simulink model "rocketSim"  (R2019a)
settings: Solver=ode3  StartTime=0.0  StopTime=t2  FixedStep=simPrm.h  MaxStep=simPrm.h  RelTol=1e-3
undefined symbols (not defined in the file or in its folder): thr
libraries: sm_lib x6, nesl_utility x6, simulink_extras x2
settings Model: Creator=vmali  LastModifiedBy=vmali
settings DebuggingCC: BusObjectLabelMismatch=none
settings SimscapeCC: SimscapeNormalizeSystem=off  SimscapeLogType=all
settings ExplorerConfigSet: InternalSimMechanicsExplorerSettings="<ExplorerConfiguration><canonicalview>default</canonicalview><AnimationSetting><BasePlaybackSpeed>1.0</BasePlaybackSpeed><PlaybackSpeedFactor>1.0</PlaybackSpeedFactor></AnimationSetting><TilePanel><TileInfo><Tiles Columns=\"1\" Count=\"1\" Rows=\"1\"><Column Weight=\"1\"/><Row Weight=\"1\"/><Tile Height=\"1\" Width=\"1\" X=\"0\" Y=\"0\"/></Tiles></TileInfo><SceneInfo><SceneViewer><BGColor><R>0.60000002384185791</R><G>0.60000002384185791</G><B>0.60000002384185791</B></BGColor><Camera><DoPerspective>off</DoPerspective><Position><X>172.69681181507903</X><Y>-34.9970129098614251</Y><Z>180.545841253777326</Z></Position><Center><X>172.518361402320892</X><Y>-34.4223760725900263</Y><Z>0.262351084401639012</Z></Center><Up><X>-0.00981184985509124183</X><Y>0.999946752141307016</Y><Z>0.00319694924480169555</Z></Up><ViewLimDist>1</ViewLimDist><YLim>132.755471146486911</YLim><XLim>205.915521409793769</XLim></Camera></SceneViewer></SceneInfo></TilePanel><MechEditorPanel><Cameras/><GfxPanelCameraMap/><VideoCreator><PlaybackSpeedRatio>1.0</PlaybackSpeedRatio><FrameRate>30</FrameRate><VideoFormat>Motion JPEG AVI</VideoFormat><FrameSize>auto</FrameSize></VideoCreator></MechEditorPanel></ExplorerConfiguration>"

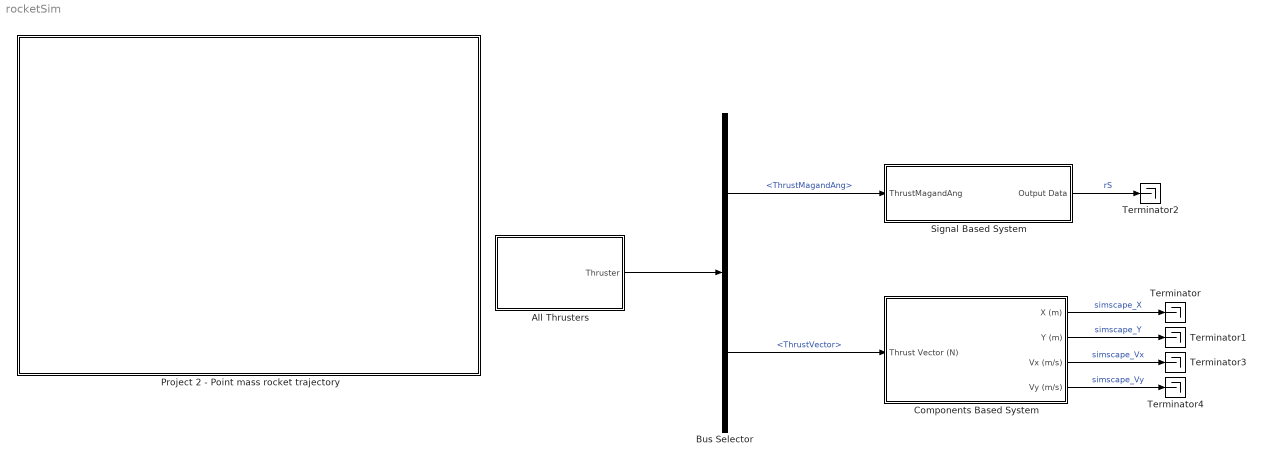
== system rocketSim ==
  All Thrusters : Subsystem
  Bus Selector : BusSelector  OutputSignals=ThrustMagandAng,ThrustVector
  Components Based System : Subsystem
  Project 2 - Point mass rocket trajectory : Subsystem
      mask Display:
      | % Use specified image as mask icon
      | image('Project2.jpg')
  Signal Based System : Subsystem
  Terminator{,1..4} (5 alike) : Terminator
  wires:
  All Thrusters/1(Thruster) -> Bus Selector/1
  Bus Selector/2 -> Components Based System/1(Thrust Vector (N))  "<ThrustVector>"
  Components Based System/1(X (m)) -> Terminator/1  "simscape_X"
  Components Based System/2(Y (m)) -> Terminator1/1  "simscape_Y"
  Bus Selector/1 -> Signal Based System/1(ThrustMagandAng)  "<ThrustMagandAng>"
  Signal Based System/1(Output Data) -> Terminator2/1  "rS"
  Components Based System/3(Vx (m/s)) -> Terminator3/1  "simscape_Vx"
  Components Based System/4(Vy (m/s)) -> Terminator4/1  "simscape_Vy"

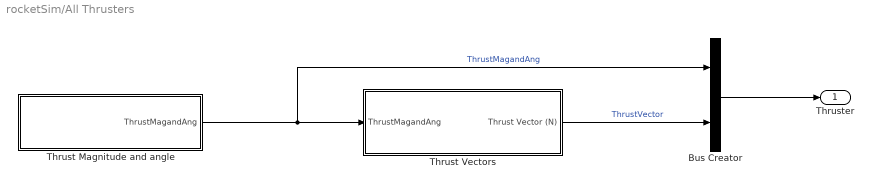
== system rocketSim/All Thrusters ==
  Bus Creator : BusCreator  Inputs=2
  Thrust Magnitude and angle : Subsystem  Variant=on
  Thrust Vectors : Subsystem
  Thruster : Outport
  wires:
  Bus Creator/1 -> Thruster/1
  Thrust Vectors/1(Thrust Vector (N)) -> Bus Creator/2  "ThrustVector"
  Thrust Magnitude and angle/1(ThrustMagandAng) -> Thrust Vectors/1(ThrustMagandAng), Bus Creator/1  "ThrustMagandAng"

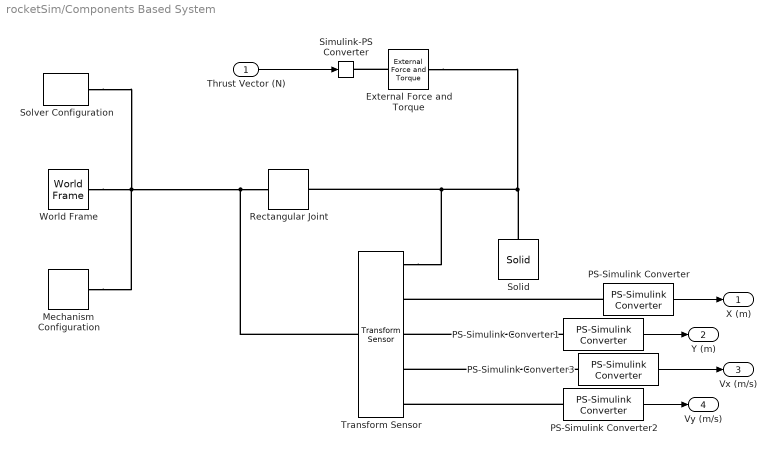
== system rocketSim/Components Based System ==
  Thrust Vector (N) : Inport
  External Force and Torque : sm_lib/Forces and Torques/External Force and Torque  ForceResolutionFrame=AttachedFrame  EnableForceX=off  EnableForceY=off  EnableForceZ=off  EnableForce=on  TorqueResolutionFrame=AttachedFrame  EnableTorqueX=off  EnableTorqueY=off  EnableTorqueZ=off  EnableTorque=off
  Mechanism Configuration : sm_lib/Utilities/Mechanism Configuration  UniformGravity=Constant  GravityVector=[0 -10.0 0]  GravityUnits=m/s^2  LinearizationDelta=0.001
  PS-Simulink Converter{,1..3} (4 alike) : nesl_utility/PS-Simulink Converter  PhysicalDomain=network_engine_domain  SubClassName=ps_output  LeftPortType=input  RightPortType=output  PseudoPeriodic=off  Frequencies=[]  Unit=1  AffineConversion=off
  Rectangular Joint : sm_lib/Joints/Rectangular Joint  SenseConstraintForce=off  SenseConstraintForceX=off  SenseConstraintForceY=off  SenseConstraintForceZ=off  SenseConstraintTorque=off  SenseConstraintTorqueX=off  SenseConstraintTorqueY=off  SenseConstraintTorqueZ=off  SenseTotalForce=off  SenseTotalForceX=off  SenseTotalForceY=off  SenseTotalForceZ=off  SenseTotalTorque=off  SenseTotalTorqueX=off  SenseTotalTorqueY=off  SenseTotalTorqueZ=off  CompositeWrenchDir=FollowerOnBase  CompositeWrenchFrame=BaseFrame  PxEquilibriumPosition=0  PxEquilibriumPositionUnits=m  PxSpringStiffness=0  PxSpringStiffnessUnits=N/m  PxDampingCoefficient=0  PxDampingCoefficientUnits=N/(m/s)  PxTorqueActuationMode=NoTorque  PxMotionActuationMode=ComputedMotion  PxSensePosition=off  PxSenseVelocity=off  PxSenseAcceleration=off  PxSenseTorqueForce=off  PxSenseLowerLimitTorqueForce=off  PxSenseUpperLimitTorqueForce=off  PxLowerLimitSpecify=off  PxLowerLimitBound=-1  PxLowerLimitBoundUnits=m  PxLowerLimitStiffness=1e6  PxLowerLimitStiffnessUnits=N/m  PxLowerLimitDamping=1e3  PxLowerLimitDampingUnits=N/(m/s)  PxLowerLimitTransitionRegionWidth=1e-4  PxLowerLimitTransitionRegionWidthUnits=m  PxUpperLimitSpecify=off  PxUpperLimitBound=1  PxUpperLimitBoundUnits=m  PxUpperLimitStiffness=1e6  PxUpperLimitStiffnessUnits=N/m  PxUpperLimitDamping=1e3  PxUpperLimitDampingUnits=N/(m/s)  PxUpperLimitTransitionRegionWidth=1e-4  PxUpperLimitTransitionRegionWidthUnits=m  PxPositionTargetSpecify=off  PxPositionTargetPriority=High  PxPositionTargetValue=0  PxPositionTargetValueUnits=m  PxVelocityTargetSpecify=off  PxVelocityTargetPriority=High  PxVelocityTargetValue=0  PxVelocityTargetValueUnits=m/s  PyEquilibriumPosition=0  PyEquilibriumPositionUnits=m  PySpringStiffness=0  PySpringStiffnessUnits=N/m  PyDampingCoefficient=0  PyDampingCoefficientUnits=N/(m/s)  PyTorqueActuationMode=NoTorque  PyMotionActuationMode=ComputedMotion  PySensePosition=off  PySenseVelocity=off  PySenseAcceleration=off  PySenseTorqueForce=off  PySenseLowerLimitTorqueForce=off  PySenseUpperLimitTorqueForce=off  PyLowerLimitSpecify=off  PyLowerLimitBound=-1  PyLowerLimitBoundUnits=m  PyLowerLimitStiffness=1e6  PyLowerLimitStiffnessUnits=N/m  PyLowerLimitDamping=1e3  PyLowerLimitDampingUnits=N/(m/s)  PyLowerLimitTransitionRegionWidth=1e-4  PyLowerLimitTransitionRegionWidthUnits=m  PyUpperLimitSpecify=off  PyUpperLimitBound=1  PyUpperLimitBoundUnits=m  PyUpperLimitStiffness=1e6  PyUpperLimitStiffnessUnits=N/m  PyUpperLimitDamping=1e3  PyUpperLimitDampingUnits=N/(m/s)  PyUpperLimitTransitionRegionWidth=1e-4  PyUpperLimitTransitionRegionWidthUnits=m  PyPositionTargetSpecify=off  PyPositionTargetPriority=High  PyPositionTargetValue=0  PyPositionTargetValueUnits=m  PyVelocityTargetSpecify=off  PyVelocityTargetPriority=High  PyVelocityTargetValue=0  PyVelocityTargetValueUnits=m/s
      settings: SourceProductName=Simscape Multibody
  Simulink-PS Converter : nesl_utility/Simulink-PS Converter  PhysicalDomain=network_engine_domain  SubClassName=ps_input  LeftPortType=input  RightPortType=output  PseudoPeriodic=off  Frequencies=[]  NoiseDistribution=none  NoiseParameters=[]  Unit=1  AffineConversion=off  FilteringAndDerivatives=provide  SimscapeFilterOrder=1  InputFilterTimeConstant=0.001  UdotUserProvided=0
  Solid : sm_lib/Body Elements/Solid  InertiaType=PointMass  Mass=1000  MassUnits=kg  CenterOfMass=[0 0 0]  CenterOfMassUnits=m  MomentsOfInertia=[1 1 1]  MomentsOfInertiaUnits=kg*m^2  ProductsOfInertia=[0 0 0]  ProductsOfInertiaUnits=kg*m^2  BasedOnType=Density  Density=1000  DensityUnits=kg/m^3  DoExposeReferenceFrame=on  SerializedFrames=<Frames/>  GraphicType=FromGeometry  MarkerShape=Sphere  MarkerSize=10  GraphicVisPropType=SimpleVisualProperties  GraphicDiffuseColor=[1.0 0.2 0.2]  GraphicSpecularColor=[0.5 0.5 0.5 1.0]  GraphicAmbientColor=[0.15 0.15 0.15 1.0]  GraphicEmissiveColor=[0.0 0.0 0.0 1.0]  GraphicShininess=75  GraphicOpacity=1.0  GeometryShape=Sphere  RectangleSize=[1 1]  RectangleSizeUnits=m  BrickDimensions=[1 1 1]  BrickDimensionUnits=m  CylinderRadius=1  CylinderRadiusUnits=m  CylinderLength=1  CylinderLengthUnits=m  SphereRadius=1  SphereRadiusUnits=m  EllipsoidRadii=[1 1 1]  EllipsoidRadiiUnits=m  ExtrusionCrossSection=[1 1; -1 1; -1 -1; 1 -1]  ExtrusionCrossSectionUnits=m  ExtrusionLength=1  ExtrusionLengthUnits=m  PolygonNumSides=3  PolygonOuterRadius=1  PolygonOuterRadiusUnits=m  ExtGeomFileType=STEP  ExtGeomFileUnits=m  RevolutionCrossSection=[1 1; 1 -1; 2 -1; 2 1]  RevolutionCrossSectionUnits=m  RevolutionExtent=Full  RevolutionAngle=180  RevolutionAngleUnits=deg
  Solver Configuration : nesl_utility/Solver Configuration  PhysicalDomain=network_engine_domain  SubClassName=solver  LeftPortType=input  RightPortType=generic  Tones=[]  Harmonics=[]  SimulateNoise=off  Profile=off  UseLocalSampling=off  EnableSwitchedLinearOptims=on  FrequencyDomain=off  UseCCode=off  RelTol=0.001  AbsTol=1e-06  MinStep=1e-09  ToWorkspace=off  RevertToSquareIcSolve=off  NumHomotopyIterations=100  PhasorMode=off  PhasorModeNumHarmonics=1  DoDC=off  ResidualTolerance=1e-09  UseLocalSolver=off  LocalSolverChoice=NE_BACKWARD_EULER_ADVANCER  LocalSolverSampleTime=0.001  DoFixedCost=off  MaxNonlinIter=3  MaxModeIter=2  LinearAlgebra=auto  EquationFormulation=NE_TIME_EF  DelaysMemoryBudget=1024  AutomaticFiltering=on  FilteringTimeConstant=0.001  PartitionStorageMethod=AS_NEEDED  PartitionMemoryBudget=1024  PartitionMethod=ROBUST
  Transform Sensor : sm_lib/Frames and Transforms/Transform Sensor  MeasurementFrame=World  SenseAngle=off  SenseAxis=off  SenseAngle1=off  SenseAngle2=off  SenseAngle3=off  SenseQ=off  SenseR=off  SenseOmegaX=off  SenseOmegaY=off  SenseOmegaZ=off  SenseOmega1=off  SenseOmega2=off  SenseOmega3=off  SenseQDot=off  SenseRDot=off  SenseAlphaX=off  SenseAlphaY=off  SenseAlphaZ=off  SenseAlpha1=off  SenseAlpha2=off  SenseAlpha3=off  SenseQDDot=off  SenseRDDot=off  SenseX=on  SenseY=on  SenseZ=off  SenseRad=off  SenseAzim=off  SenseDist=off  SenseInc=off  SenseXDot=on  SenseYDot=on  SenseZDot=off  SenseRadDot=off  SenseAzimDot=off  SenseDistDot=off  SenseIncDot=off  SenseXDDot=off  SenseYDDot=off  SenseZDDot=off  SenseRadDDot=off  SenseAzimDDot=off  SenseDistDDot=off  SenseIncDDot=off
  World Frame : sm_lib/Frames and Transforms/World Frame
  X (m) : Outport
  Y (m) : Outport  Port=2
  Vx (m/s) : Outport  Port=3
  Vy (m/s) : Outport  Port=4
  wires:
  Thrust Vector (N)/1 -> Simulink-PS Converter/1
  PS-Simulink Converter/1 -> X (m)/1
  PS-Simulink Converter1/1 -> Y (m)/1
  PS-Simulink Converter2/1 -> Vy (m/s)/1
  PS-Simulink Converter3/1 -> Vx (m/s)/1
  connections:
  World Frame/RConn1 -- Mechanism Configuration/RConn1 -- Solver Configuration/RConn1 -- Transform Sensor/LConn1 -- Rectangular Joint/LConn1
  Solid/RConn1 -- External Force and Torque/RConn1 -- Transform Sensor/RConn1 -- Rectangular Joint/RConn1
  External Force and Torque/LConn1 -- Simulink-PS Converter/RConn1
  PS-Simulink Converter/LConn1 -- Transform Sensor/RConn2
  PS-Simulink Converter1/LConn1 -- Transform Sensor/RConn3
  PS-Simulink Converter2/LConn1 -- Transform Sensor/RConn5
  PS-Simulink Converter3/LConn1 -- Transform Sensor/RConn4

== system rocketSim/Project 2 - Point mass rocket trajectory ==

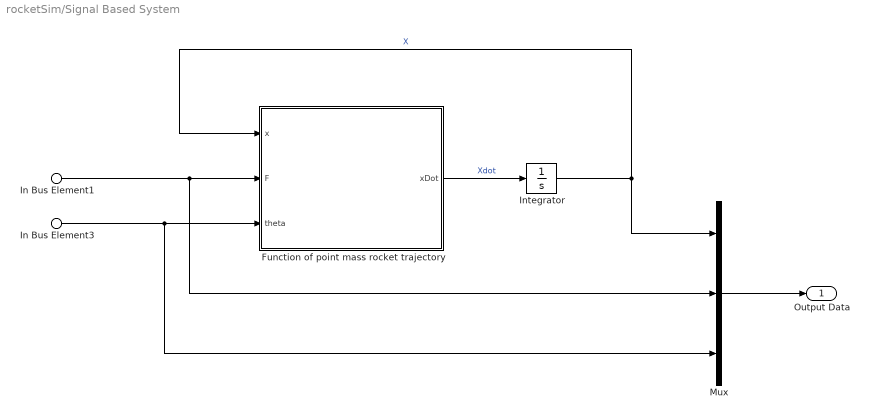
== system rocketSim/Signal Based System ==
  In Bus Element1 : Inport  PortName=ThrustMagandAng  Element=Magnitude
  In Bus Element3 : Inport  PortName=ThrustMagandAng  Element=Angle
  Function of point mass rocket trajectory : MATLAB Function  TreatAsAtomicUnit=on
  Integrator : Integrator
  Mux : Mux  Inputs=3
  Output Data : Outport
  wires:
  Function of point mass rocket trajectory/1(xDot) -> Integrator/1  "Xdot"
  Integrator/1 -> Mux/1, Function of point mass rocket trajectory/1(x)  "X"
  In Bus Element1/1 -> Mux/2, Function of point mass rocket trajectory/2(F)
  In Bus Element3/1 -> Mux/3, Function of point mass rocket trajectory/3(theta)
  Mux/1 -> Output Data/1

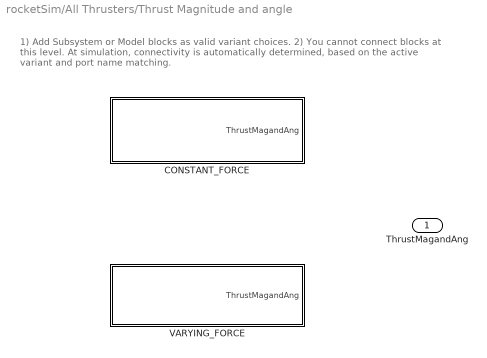
== system rocketSim/All Thrusters/Thrust Magnitude and angle ==
  note: 1) Add Subsystem or Model blocks as valid variant choices.
      | 2) You cannot connect blocks at this level. At simulation, connectivity is automatically
      | determined, based on the active variant and port name matching.
  CONSTANT_FORCE : Subsystem  Description=This is the block containing the constant thrust value.  VariantControl=CONSTANT_F_VSS
  VARYING_FORCE : Subsystem  Description=This is the block containing the constant thrust value.  VariantControl=VARYING_F_VSS
  ThrustMagandAng : Outport

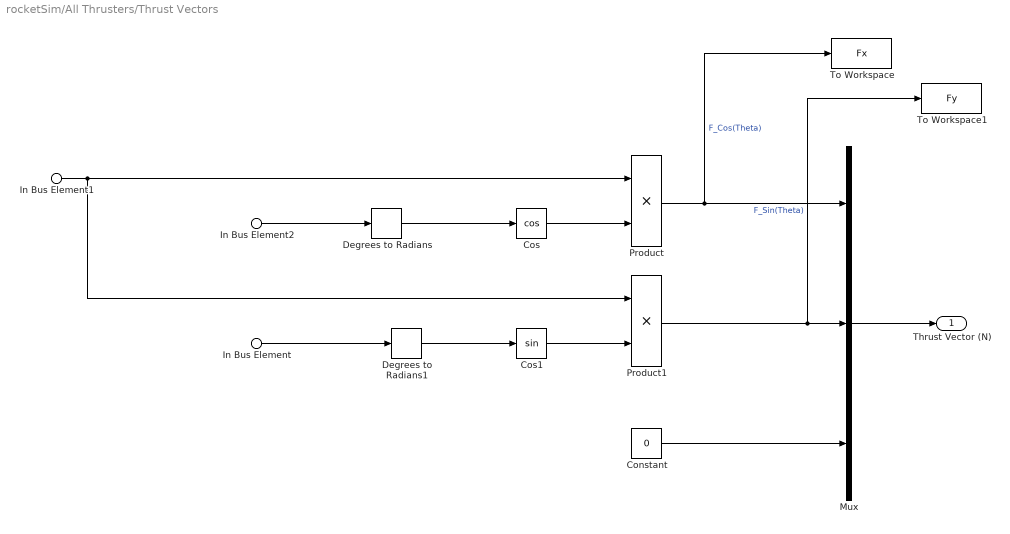
== system rocketSim/All Thrusters/Thrust Vectors ==
  In Bus Element1 : Inport  PortName=ThrustMagandAng  Element=Magnitude
  In Bus Element2 : Inport  PortName=ThrustMagandAng  Element=Angle
  In Bus Element : Inport  PortName=ThrustMagandAng  Element=Angle
  Constant : Constant  Value=0
  Cos : Trigonometry  Operator=cos
  Cos1 : Trigonometry
  Degrees to Radians : simulink_extras/Transformations/Degrees to Radians
  Degrees to Radians1 : simulink_extras/Transformations/Degrees to Radians
  Mux : Mux  Inputs=3
  Product : Product
  Product1 : Product
  To Workspace : ToWorkspace  VariableName=Fx  SaveFormat=Timeseries  SampleTime=-1
  To Workspace1 : ToWorkspace  VariableName=Fy  SaveFormat=Timeseries  SampleTime=-1
  Thrust Vector (N) : Outport
  wires:
  In Bus Element2/1 -> Degrees to Radians/1
  Cos/1 -> Product/2
  In Bus Element/1 -> Degrees to Radians1/1
  In Bus Element1/1 -> Product1/1, Product/1
  Cos1/1 -> Product1/2
  Product/1 -> To Workspace/1, Mux/1  "F_Cos(Theta)"
  Product1/1 -> To Workspace1/1, Mux/2  "F_Sin(Theta)"
  Constant/1 -> Mux/3
  Mux/1 -> Thrust Vector (N)/1
  Degrees to Radians/1 -> Cos/1
  Degrees to Radians1/1 -> Cos1/1

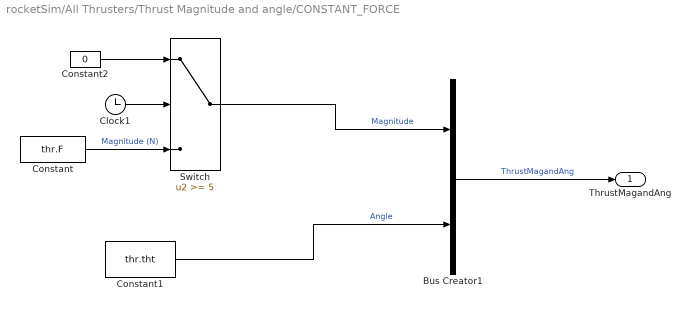
== system rocketSim/All Thrusters/Thrust Magnitude and angle/CONSTANT_FORCE ==
  Bus Creator1 : BusCreator  Inputs=2
  Clock1 : Clock
  Constant : Constant  Value=thr.F
  Constant1 : Constant  Value=thr.tht
  Constant2 : Constant  Value=0
  Switch : Switch  Threshold=5
  ThrustMagandAng : Outport  OutDataTypeStr=Bus: Scenario_1
  wires:
  Constant1/1 -> Bus Creator1/2  "Angle"
  Clock1/1 -> Switch/2
  Constant2/1 -> Switch/1
  Constant/1 -> Switch/3  "Magnitude (N)"
  Switch/1 -> Bus Creator1/1  "Magnitude"
  Bus Creator1/1 -> ThrustMagandAng/1  "ThrustMagandAng"

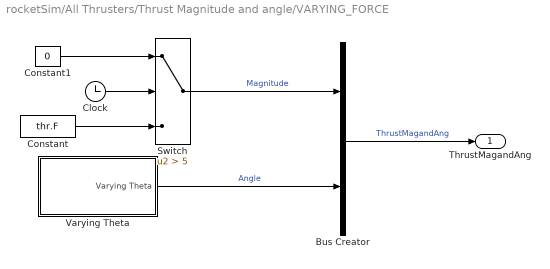
== system rocketSim/All Thrusters/Thrust Magnitude and angle/VARYING_FORCE ==
  Bus Creator : BusCreator  Inputs=2
  Clock : Clock
  Constant : Constant  Value=thr.F
  Constant1 : Constant  Value=0
  Switch : Switch  Criteria=u2 > Threshold  Threshold=5
  Varying Theta : Subsystem
  ThrustMagandAng : Outport  OutDataTypeStr=Bus: Scenario_2
  wires:
  Varying Theta/1(Varying Theta) -> Bus Creator/2  "Angle"
  Bus Creator/1 -> ThrustMagandAng/1  "ThrustMagandAng"
  Constant1/1 -> Switch/1
  Constant/1 -> Switch/3
  Switch/1 -> Bus Creator/1  "Magnitude"
  Clock/1 -> Switch/2

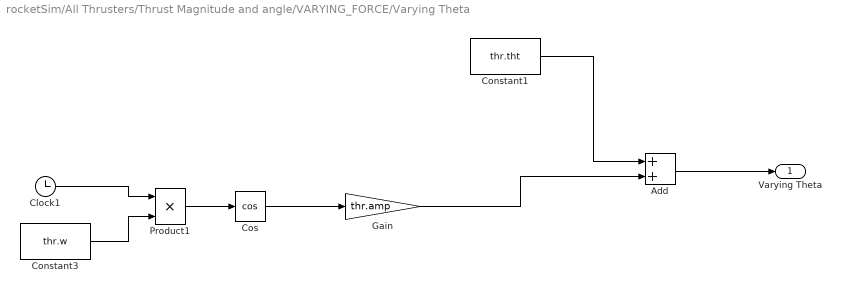
== system rocketSim/All Thrusters/Thrust Magnitude and angle/VARYING_FORCE/Varying Theta ==
  Add : Sum
  Clock1 : Clock
  Constant1 : Constant  Value=thr.tht
  Constant3 : Constant  Value=thr.w
  Cos : Trigonometry  Operator=cos
  Gain : Gain  Gain=thr.amp
  Product1 : Product
  Varying Theta : Outport
  wires:
  Gain/1 -> Add/2
  Constant1/1 -> Add/1
  Add/1 -> Varying Theta/1
  Product1/1 -> Cos/1
  Constant3/1 -> Product1/2
  Clock1/1 -> Product1/1
  Cos/1 -> Gain/1

== matlab function rocketSim/Signal Based System/Function of point mass rocket trajectory ==
  data: x input; xDot output; F input; theta input
function xDot = f(x,F, theta)
% Function f of x' = f(x)
% x == states

%Give the input parameters

m = 1000;  % mass of roket in kg
g = 10;    % Physical constant - grav. acceleration

% grab memory
xDot = zeros(4,1);

% fill in f of x' = f(x)
xDot(1) = x(3);  % Velocity in X direction
xDot(2) = x(4);  % Velocity in Y direction
xDot(3) = (F/m)*cosd(theta);  % Acceleration in X direction
xDot(4) = (F/m)*sind(theta)- g;  % Acceleration in Y direction
